simulink model "blockDiagramTask6"  (R2025a)
settings: Solver=VariableStepAuto  StartTime=0.0  StopTime=3.10  RelTol=1e-3
InitFcn:
  | run motor_specs.m
model workspace: external: MATLAB File motor_specs.m (data not in the file)
values from neighbouring files (symbols this model uses):
  A6 = [zeros(2) E; ((-inv(inertiaMatrix)) * stiffnessMatrix), ((-inv(inertiaMatrix)) * dampingMatrix)]    [ssAndTF.m]
  B6 = [zeros(2) inv(inertiaMatrix)]'    [ssAndTF.m]
  C6 = [0 1 0 0]    [ssAndTF.m]
  d_j = 1.5    [motor_specs.m]
  K_E = 0.006741/rpm_to_rs    (= 0.0643718082829)    [motor_specs.m]
  R = 3.23    [motor_specs.m]
  totalGearRatio = torqueSection2 / (torqueSection1 * totalEfficiency)    [ssAndTF.m]
  U_N = 36    [motor_specs.m]
undefined symbols (not defined in the file or in its folder): A8, delta_ratio, k_j, k_theta, my, r_s, sigbuilder_block, T_thresh_2
libraries: slpidlib x3
settings Model: Creator=josef  LastModifiedBy=lucas

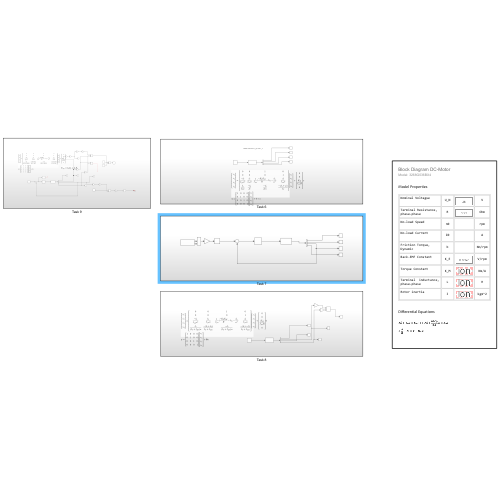
[thumbnail: Simulink's stored preview of the top-level diagram]
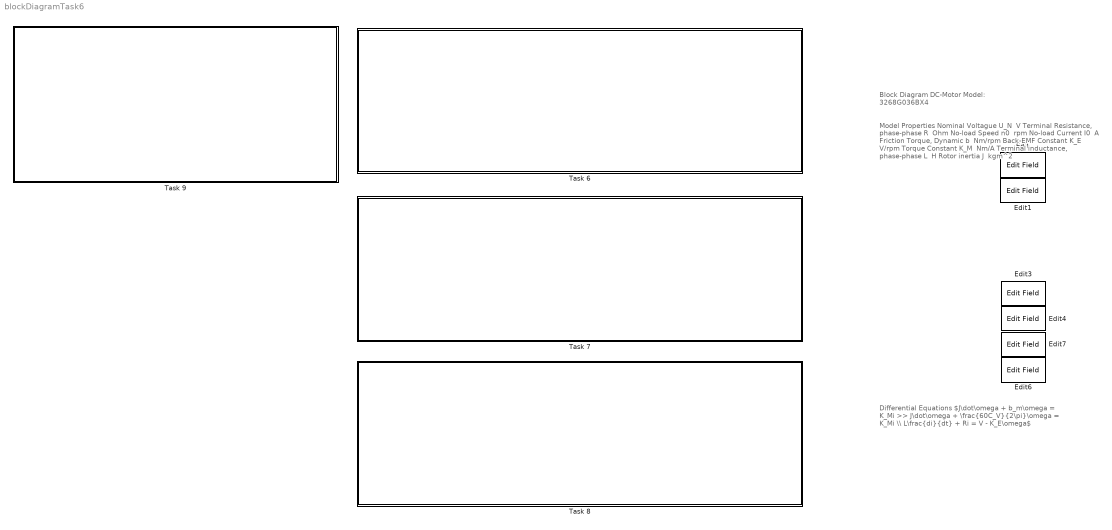
== system blockDiagramTask6 ==
  note: Differential Equations
      |
      | $J\dot\omega + b_m\omega = K_Mi >> J\dot\omega + \frac{60C_V}{2\pi}\omega = K_Mi \\ L\frac{di}{dt} + Ri = V - K_E\omega$
  note: Model Properties
      |
      | Nominal Voltague
      |
      | U_N
      | ​
      | V
      |
      | Terminal Resistance,
      | phase-phase
      | R
      | ​
      | Ohm
      |
      | No-load Speed
      |
      | n0
      | ​
      | rpm
      |
      | No-load Current
      |
      | I0
      | ​
      | A
      |
      | Friction Torque,
      | Dynamic
      | b
      | ​
      | Nm/rpm
      |
      | Back-EMF Constant
      |
      | K_E
      | ​
      | V/rpm
      |
      | Torque Constant
      |
      | K_M
      | ​
      | Nm/A
      |
      | Terminal inductance,
      | phase-phase
      | L
      | ​
      | H
      |
      | Rotor inertia
      |
      | J
      | ​
      | kgm^2
  note: Block Diagram DC-Motor
      | Model: 3268G036BX4
  Edit{,1,3..4,6..7} (6 alike) : EditField  LabelPosition=Hide  ShowInitialText=on  Alignment=Center  Opacity=0
  Task 6 : Subsystem
  Task 7 : Subsystem
  Task 8 : Subsystem
  Task 9 : Subsystem

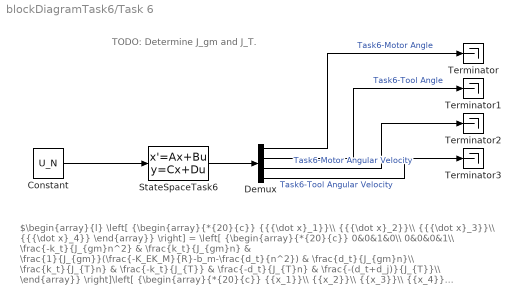
== system blockDiagramTask6/Task 6 ==
  note: TODO: Determine J_gm and J_T.
  note: $\begin{array}{l} \left[ {\begin{array}{*{20}{c}} {{{\dot x}_1}}\\ {{{\dot x}_2}}\\ {{{\dot x}_3}}\\ {{{\dot x}_4}} \end{array}} \right] = \left[ {\begin{array}{*{20}{c}} 0&0&1&0\\ 0&0&0&1\\ \frac{-k_t}{J_{gm}n^2} & \frac{k_t}{J_{gm}n} & \frac{1}{J_{gm}}(\frac{-K_EK_M}{R}-b_m-\frac{d_t}{n^2}) & \frac{d_t}{J_{gm}n}\\ \frac{k_t}{J_{T}n} & \frac{-k_t}{J_{T}} & \frac{-d_t}{J_{T}n} & \frac{-(d_t+d_j)}{J_{T}}\\ \end{array}} \right]\left[ {\begin{array}{*{20}{c}} {{x_1}}\\ {{x_2}}\\ {{x_3}}\\ {{x_4}} \end{array}} \right] + \left[ {\begin{array}{*{20}{c}} 0\\ 0\\ \frac{K_M}{J_{gm}R} \\ 0 \\ \end{array}} \right]u\\ {\bf{y}} = \left[ {\begin{array}{*{20}{c}} 1&0&0&0\\ 0&1&0&0\\ 0&0&1&0\\ 0&0&0&1\\ \end{array}} \right]\left[ {\begin{array}{*{20}{c}} {{x_1}}\\ {{x_2}}\\ {{x_3}}\\ {{x_4}} \end{array}} \right] + 0*u \end{array}$
  Constant : Constant  Value=U_N
  Demux : Demux
  StateSpaceTask6 : StateSpace  A=A6  B=B6  C=C6  D=[0;0;0;0]  InitialCondition=0
  Terminator{,1..3} (4 alike) : Terminator
  wires:
  StateSpaceTask6/1 -> Demux/1
  Demux/1 -> Terminator/1  "Task6-Motor Angle"
  Demux/2 -> Terminator1/1  "Task6-Tool Angle"
  Demux/3 -> Terminator2/1  "Task6-Motor Angular Velocity"
  Demux/4 -> Terminator3/1  "Task6-Tool Angular Velocity"
  Constant/1 -> StateSpaceTask6/1

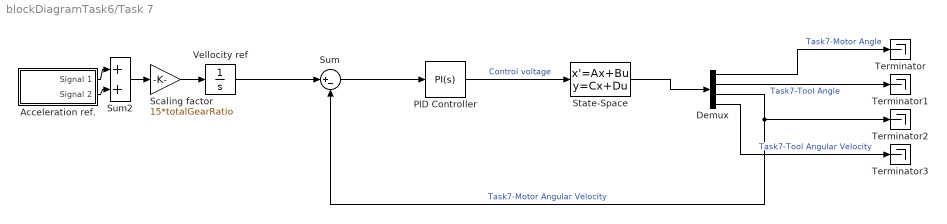
== system blockDiagramTask6/Task 7 ==
  Acceleration ref. : Subsystem  Tag=STV Subsys  LoadFcn=sigbuilder_block('load');  StartFcn=sigbuilder_block('start');  StopFcn=sigbuilder_block('stop');  ClipboardFcn=sigbuilder_block('clipboard');  mask(Sigbuilder block){tuvar=[0:10]}
      mask help: Sigbuilder GUI
      mask init:
      | if ~strcmp(get_param(bdroot(gcbh),'SimulationStatus'),'stopped') tuvar = sigbuilder_block('maskInit'); end
      settings: CopyFcn=sigbuilder_block('copy');  DeleteFcn=sigbuilder_block('delete');  ModelCloseFcn=sigbuilder_block('modelClose');  PreSaveFcn=sigbuilder_block('preSave');  PauseFcn=sigbuilder_block('pause')  ContinueFcn=sigbuilder_block('continue')  NameChangeFcn=sigbuilder_block('namechange');  OpenFcn=sigbuilder_block('open',[210.75 63.75 537 323.25 ]);  CloseFcn=sigbuilder_block('close');
      mask Display: plot(0, 0, 100, 100,[2, 2, 32, 32, 2], [68, 8, 8, 68, 68],[32, 2], [38, 38], [32, 19, 2],[53, 60, 44], [32, 17, 17, 2],[16, 16, 31, 31]);txt = getActiveGroup(gcbh);text(2, 100, txt,'verticalAlignment', 'top');
  Demux : Demux
  PID Controller : slpidlib/PID Controller  Controller=PI  Form=Parallel  TimeDomain=Continuous-time  UseExternalTs=off  SampleTime=-1  IntegratorMethod=Forward Euler  FilterMethod=Forward Euler  ControllerParametersSource=internal  P=0.589073731906208  I=155.603114436522  UseKiTs=off  D=0  UseExternalDerivativeSource=off  N=100  UseFilter=on  TunerSelectOption=Transfer Function Based (PID Tuner App)  InitialConditionSource=internal  InitialConditionForIntegrator=0  InitialConditionForFilter=0  DifferentiatorICPrevScaledInput=0  ExternalReset=none  TrackingMode=off  Kt=1  LimitOutput=off  SatLimitsSource=internal  UpperSaturationLimit=inf  LowerSaturationLimit=-inf  LinearizeAsGain=on  AntiWindupMode=none  Kb=1  LimitIntegrator=off  UpperIntegratorSaturationLimit=inf  LowerIntegratorSaturationLimit=-inf  POutMin=[]  POutMax=[]  IOutMin=[]  IOutMax=[]  DOutMin=[]  DOutMax=[]  NOutMin=[]  NOutMax=[]  SumOutMin=[]  SumOutMax=[]  SaturationOutMin=[]  SaturationOutMax=[]  PParamMin=[]  PParamMax=[]  IParamMin=[]  IParamMax=[]  DParamMin=[]  DParamMax=[]  NParamMin=[]  NParamMax=[]  KbParamMin=[]  KbParamMax=[]  KtParamMin=[]  KtParamMax=[]  KbOutMin=[]  KbOutMax=[]  KtOutMin=[]  KtOutMax=[]  IntegratorOutMin=[]  IntegratorOutMax=[]  FilterOutMin=[]  FilterOutMax=[]  SumI1OutMin=[]  SumI1OutMax=[]  SumI2OutMin=[]  SumI2OutMax=[]  SumI3OutMin=[]  SumI3OutMax=[]  SumI4OutMin=[]  SumI4OutMax=[]  SumDOutMin=[]  SumDOutMax=[]  DifferentiatorOutMin=[]  DifferentiatorOutMax=[]  FilterDiffOutCoefMin=[]  FilterDiffOutCoefMax=[]  ReciprocalOutMin=[]  ReciprocalOutMax=[]  SumDenOutMin=[]  SumDenOutMax=[]  SumNumOutMin=[]  SumNumOutMax=[]  DivideOutMin=[]  DivideOutMax=[]  UdiffTsProdOutMin=[]  UdiffTsProdOutMax=[]  NTsProdOutMin=[]  NTsProdOutMax=[]  UintegralTsProdOutMin=[]  UintegralTsProdOutMax=[]  UngainTsProdOutMin=[]  UngainTsProdOutMax=[]  ClampingZeroOutDataTypeStr=Inherit: Inherit via back propagation  ClampingZeroOutMin=[]  ClampingZeroOutMax=[]  FilterDenConstantOutDataTypeStr=Inherit: Inherit via back propagation  FilterDenConstantOutMin=[]  FilterDenConstantOutMax=[]  PCopyOutDataTypeStr=Inherit: Inherit via back propagation  PCopyOutMin=[]  PCopyOutMax=[]  NCopyOutDataTypeStr=Inherit: Inherit via back propagation  NCopyOutMin=[]  NCopyOutMax=[]  IntegratorContinuousStateAttributes=''  IntegratorStateMustResolveToSignalObject=off  IntegratorRTWStateStorageClass=Auto  FilterContinuousStateAttributes=''  FilterStateMustResolveToSignalObject=off  FilterRTWStateStorageClass=Auto  ParallelPVariant=InternalParameters  IdealPVariant=Disabled  IVariant=InternalParameters  DVariant=Disabled  IntegratorVariant=Continuous  SatVariant=Disabled  AWVariant=Passthrough  PCopyVariant=Disabled  TRVariant=Disabled  FdbkBlocksVariant=Forward  IdealPFdbkVariant=Disabled  SatFdbkVariant=Disabled  DerivativeFilterVariant=Disabled  NVariant=Disabled  NCopyVariant=Disabled_SignalSpec  FilterICVariant=Disabled  IntegratorICVariant=InternalICs  ExternalResetVariant=Disabled  TRSumVariant=Passthrough  SumFdbkVariant=Disabled  SumVariant=Sum_PI  TsampFilterVariant=InternalTs  TsampNgainVariant=Passthrough  TsampIntegralVariant=Disabled_SignalSpec  ExternalSaturationOutDataTypeStr=Inherit: Same as second input  DerivativeSourceVariant=Disabled  PreIntVariant=InternalPreInt
  Scaling factor : Gain  Gain=15*totalGearRatio
  State-Space : StateSpace  A=A6  B=B6  C=C6  D=[0;0;0;0]  InitialCondition=0
  Sum : Sum  Inputs=|+-
  Sum2 : Sum  Inputs=|++
  Terminator{,1..3} (4 alike) : Terminator
  Vellocity ref : Integrator
  wires:
  PID Controller/1 -> State-Space/1  "Control voltage"
  State-Space/1 -> Demux/1
  Demux/1 -> Terminator/1  "Task7-Motor Angle"
  Demux/3 -> Sum/2, Terminator2/1  "Task7-Motor Angular Velocity"
  Demux/4 -> Terminator3/1  "Task7-Tool Angular Velocity"
  Acceleration ref./1(Signal 1) -> Sum2/1
  Acceleration ref./2(Signal 2) -> Sum2/2
  Sum2/1 -> Scaling factor/1
  Scaling factor/1 -> Vellocity ref/1
  Vellocity ref/1 -> Sum/1
  Demux/2 -> Terminator1/1  "Task7-Tool Angle"
  Sum/1 -> PID Controller/1

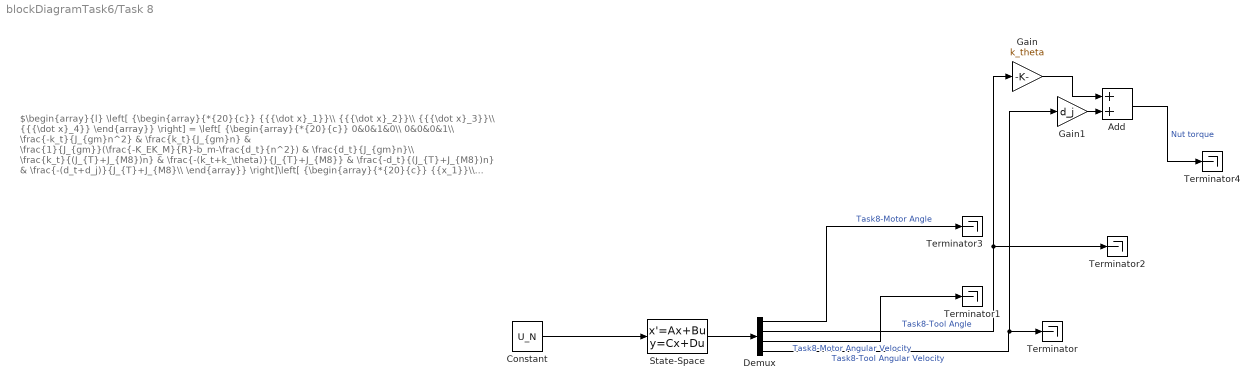
== system blockDiagramTask6/Task 8 ==
  note: $\begin{array}{l} \left[ {\begin{array}{*{20}{c}} {{{\dot x}_1}}\\ {{{\dot x}_2}}\\ {{{\dot x}_3}}\\ {{{\dot x}_4}} \end{array}} \right] = \left[ {\begin{array}{*{20}{c}} 0&0&1&0\\ 0&0&0&1\\ \frac{-k_t}{J_{gm}n^2} & \frac{k_t}{J_{gm}n} & \frac{1}{J_{gm}}(\frac{-K_EK_M}{R}-b_m-\frac{d_t}{n^2}) & \frac{d_t}{J_{gm}n}\\ \frac{k_t}{(J_{T}+J_{M8})n} & \frac{-(k_t+k_\theta)}{J_{T}+J_{M8}} & \frac{-d_t}{(J_{T}+J_{M8})n} & \frac{-(d_t+d_j)}{J_{T}+J_{M8}\\ \end{array}} \right]\left[ {\begin{array}{*{20}{c}} {{x_1}}\\ {{x_2}}\\ {{x_3}}\\ {{x_4}} \end{array}} \right] + \left[ {\begin{array}{*{20}{c}} 0\\ 0\\ \frac{K_M}{J_{gm}R}\\ 0\\ \end{array}} \right]0\\ {\bf{y}} = \left[ {\begin{array}{*{20}{c}} 1&0&0&0\\ 0&1&0&0\\ 0&0&1&0\\ 0&0&0&1\\ \end{array}} \right]\left[ {\begin{array}{*{20}{c}} {{x_1}}\\ {{x_2}}\\ {{x_3}}\\ {{x_4}} \end{array}} \right] + {\bf{0}}u \end{array}$
  Add : Sum
  Constant : Constant  Value=U_N
  Demux : Demux
  Gain : Gain  Gain=k_theta
  Gain1 : Gain  Gain=d_j
  State-Space : StateSpace  A=A8  B=B6  C=C6  D=[0;0;0;0]  InitialCondition=0
  Terminator{,1..4} (5 alike) : Terminator
  wires:
  Constant/1 -> State-Space/1
  State-Space/1 -> Demux/1
  Demux/1 -> Terminator3/1  "Task8-Motor Angle"
  Demux/2 -> Gain/1, Terminator2/1  "Task8-Tool Angle"
  Demux/3 -> Terminator1/1  "Task8-Motor Angular Velocity"
  Demux/4 -> Gain1/1, Terminator/1  "Task8-Tool Angular Velocity"
  Gain1/1 -> Add/2
  Gain/1 -> Add/1
  Add/1 -> Terminator4/1  "Nut torque"

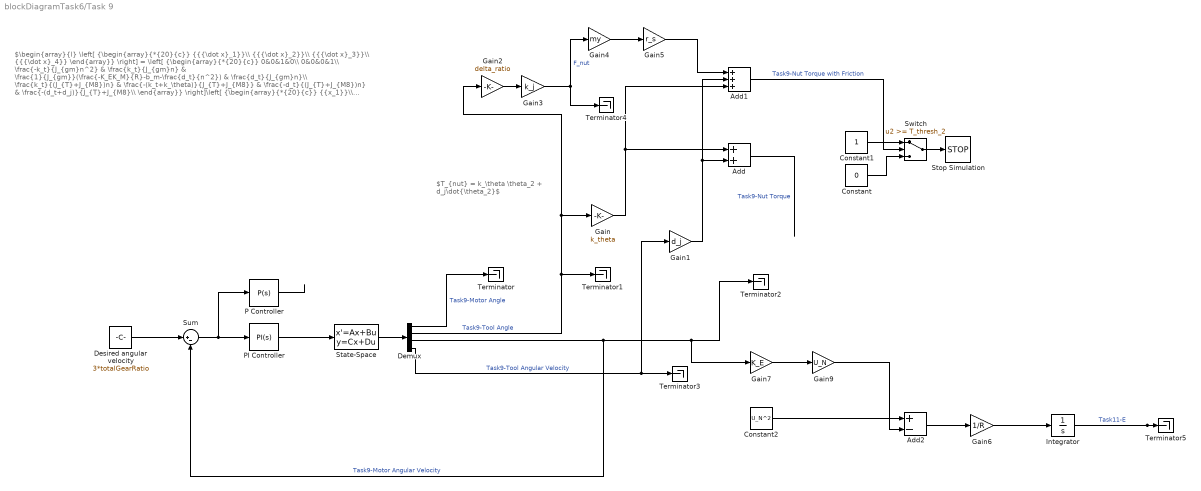
== system blockDiagramTask6/Task 9 ==
  note: $\begin{array}{l} \left[ {\begin{array}{*{20}{c}} {{{\dot x}_1}}\\ {{{\dot x}_2}}\\ {{{\dot x}_3}}\\ {{{\dot x}_4}} \end{array}} \right] = \left[ {\begin{array}{*{20}{c}} 0&0&1&0\\ 0&0&0&1\\ \frac{-k_t}{J_{gm}n^2} & \frac{k_t}{J_{gm}n} & \frac{1}{J_{gm}}(\frac{-K_EK_M}{R}-b_m-\frac{d_t}{n^2}) & \frac{d_t}{J_{gm}n}\\ \frac{k_t}{(J_{T}+J_{M8})n} & \frac{-(k_t+k_\theta)}{J_{T}+J_{M8}} & \frac{-d_t}{(J_{T}+J_{M8})n} & \frac{-(d_t+d_j)}{J_{T}+J_{M8}\\ \end{array}} \right]\left[ {\begin{array}{*{20}{c}} {{x_1}}\\ {{x_2}}\\ {{x_3}}\\ {{x_4}} \end{array}} \right] + \left[ {\begin{array}{*{20}{c}} 0\\ 0\\ \frac{K_M}{J_{gm}R}\\ 0 \\ \end{array}} \right]u\\ {\bf{y}} = \left[ {\begin{array}{*{20}{c}} 1&0&0&0\\ 0&1&0&0\\ 0&0&1&0\\ 0&0&0&1\\ \end{array}} \right]\left[ {\begin{array}{*{20}{c}} {{x_1}}\\ {{x_2}}\\ {{x_3}}\\ {{x_4}} \end{array}} \right] + {\bf{0}}u \end{array}$
  note: $T_{nut} = k_\theta \theta_2 + d_j\dot{\theta_2}$
  Add : Sum
  Add1 : Sum  Inputs=+++
  Add2 : Sum  Inputs=+-
  Constant : Constant  Value=0
  Constant1 : Constant
  Constant2 : Constant  Value=U_N^2
  Demux : Demux
  Desired angular velocity : Constant  Value=3*totalGearRatio
  Gain : Gain  Gain=k_theta
  Gain1 : Gain  Gain=d_j
  Gain2 : Gain  Gain=delta_ratio
  Gain3 : Gain  Gain=k_j
  Gain4 : Gain  Gain=my
  Gain5 : Gain  Gain=r_s
  Gain6 : Gain  Gain=1/R
  Gain7 : Gain  Gain=K_E
  Gain9 : Gain  Gain=U_N
  Integrator : Integrator
  P Controller : slpidlib/PID Controller  Controller=P  Form=Parallel  TimeDomain=Continuous-time  UseExternalTs=off  SampleTime=-1  IntegratorMethod=Forward Euler  FilterMethod=Forward Euler  ControllerParametersSource=internal  P=1  I=1  UseKiTs=off  D=0  UseExternalDerivativeSource=off  N=100  UseFilter=on  TunerSelectOption=Transfer Function Based (PID Tuner App)  InitialConditionSource=internal  InitialConditionForIntegrator=0  InitialConditionForFilter=0  DifferentiatorICPrevScaledInput=0  ExternalReset=none  TrackingMode=off  Kt=1  LimitOutput=off  SatLimitsSource=internal  UpperSaturationLimit=inf  LowerSaturationLimit=-inf  LinearizeAsGain=on  AntiWindupMode=none  Kb=1  LimitIntegrator=off  UpperIntegratorSaturationLimit=inf  LowerIntegratorSaturationLimit=-inf  POutMin=[]  POutMax=[]  IOutMin=[]  IOutMax=[]  DOutMin=[]  DOutMax=[]  NOutMin=[]  NOutMax=[]  SumOutMin=[]  SumOutMax=[]  SaturationOutMin=[]  SaturationOutMax=[]  PParamMin=[]  PParamMax=[]  IParamMin=[]  IParamMax=[]  DParamMin=[]  DParamMax=[]  NParamMin=[]  NParamMax=[]  KbParamMin=[]  KbParamMax=[]  KtParamMin=[]  KtParamMax=[]  KbOutMin=[]  KbOutMax=[]  KtOutMin=[]  KtOutMax=[]  IntegratorOutMin=[]  IntegratorOutMax=[]  FilterOutMin=[]  FilterOutMax=[]  SumI1OutMin=[]  SumI1OutMax=[]  SumI2OutMin=[]  SumI2OutMax=[]  SumI3OutMin=[]  SumI3OutMax=[]  SumI4OutMin=[]  SumI4OutMax=[]  SumDOutMin=[]  SumDOutMax=[]  DifferentiatorOutMin=[]  DifferentiatorOutMax=[]  FilterDiffOutCoefMin=[]  FilterDiffOutCoefMax=[]  ReciprocalOutMin=[]  ReciprocalOutMax=[]  SumDenOutMin=[]  SumDenOutMax=[]  SumNumOutMin=[]  SumNumOutMax=[]  DivideOutMin=[]  DivideOutMax=[]  UdiffTsProdOutMin=[]  UdiffTsProdOutMax=[]  NTsProdOutMin=[]  NTsProdOutMax=[]  UintegralTsProdOutMin=[]  UintegralTsProdOutMax=[]  UngainTsProdOutMin=[]  UngainTsProdOutMax=[]  ClampingZeroOutDataTypeStr=Inherit: Inherit via back propagation  ClampingZeroOutMin=[]  ClampingZeroOutMax=[]  FilterDenConstantOutDataTypeStr=Inherit: Inherit via back propagation  FilterDenConstantOutMin=[]  FilterDenConstantOutMax=[]  PCopyOutDataTypeStr=Inherit: Inherit via back propagation  PCopyOutMin=[]  PCopyOutMax=[]  NCopyOutDataTypeStr=Inherit: Inherit via back propagation  NCopyOutMin=[]  NCopyOutMax=[]  IntegratorContinuousStateAttributes=''  IntegratorStateMustResolveToSignalObject=off  IntegratorRTWStateStorageClass=Auto  FilterContinuousStateAttributes=''  FilterStateMustResolveToSignalObject=off  FilterRTWStateStorageClass=Auto  ParallelPVariant=InternalParameters  IdealPVariant=Disabled  IVariant=Disabled  DVariant=Disabled  IntegratorVariant=Disabled  SatVariant=Disabled  AWVariant=Disabled  PCopyVariant=Disabled  TRVariant=Disabled  FdbkBlocksVariant=Forward  IdealPFdbkVariant=Disabled  SatFdbkVariant=Disabled  DerivativeFilterVariant=Disabled  NVariant=Disabled  NCopyVariant=Disabled_SignalSpec  FilterICVariant=Disabled  IntegratorICVariant=Disabled  ExternalResetVariant=Disabled  TRSumVariant=Passthrough  SumFdbkVariant=Disabled  SumVariant=Passthrough_P  TsampFilterVariant=InternalTs  TsampNgainVariant=Passthrough  TsampIntegralVariant=Disabled_SignalSpec  ExternalSaturationOutDataTypeStr=Inherit: Same as second input  DerivativeSourceVariant=Disabled  PreIntVariant=InternalPreInt
  PI Controller : slpidlib/PID Controller  Controller=PI  Form=Parallel  TimeDomain=Continuous-time  UseExternalTs=off  SampleTime=-1  IntegratorMethod=Forward Euler  FilterMethod=Forward Euler  ControllerParametersSource=internal  P=0  I=13.2590415102096  UseKiTs=off  D=0  UseExternalDerivativeSource=off  N=100  UseFilter=on  TunerSelectOption=Transfer Function Based (PID Tuner App)  InitialConditionSource=internal  InitialConditionForIntegrator=0  InitialConditionForFilter=0  DifferentiatorICPrevScaledInput=0  ExternalReset=none  TrackingMode=off  Kt=1  LimitOutput=off  SatLimitsSource=internal  UpperSaturationLimit=inf  LowerSaturationLimit=-inf  LinearizeAsGain=on  AntiWindupMode=none  Kb=1  LimitIntegrator=off  UpperIntegratorSaturationLimit=inf  LowerIntegratorSaturationLimit=-inf  POutMin=[]  POutMax=[]  IOutMin=[]  IOutMax=[]  DOutMin=[]  DOutMax=[]  NOutMin=[]  NOutMax=[]  SumOutMin=[]  SumOutMax=[]  SaturationOutMin=[]  SaturationOutMax=[]  PParamMin=[]  PParamMax=[]  IParamMin=[]  IParamMax=[]  DParamMin=[]  DParamMax=[]  NParamMin=[]  NParamMax=[]  KbParamMin=[]  KbParamMax=[]  KtParamMin=[]  KtParamMax=[]  KbOutMin=[]  KbOutMax=[]  KtOutMin=[]  KtOutMax=[]  IntegratorOutMin=[]  IntegratorOutMax=[]  FilterOutMin=[]  FilterOutMax=[]  SumI1OutMin=[]  SumI1OutMax=[]  SumI2OutMin=[]  SumI2OutMax=[]  SumI3OutMin=[]  SumI3OutMax=[]  SumI4OutMin=[]  SumI4OutMax=[]  SumDOutMin=[]  SumDOutMax=[]  DifferentiatorOutMin=[]  DifferentiatorOutMax=[]  FilterDiffOutCoefMin=[]  FilterDiffOutCoefMax=[]  ReciprocalOutMin=[]  ReciprocalOutMax=[]  SumDenOutMin=[]  SumDenOutMax=[]  SumNumOutMin=[]  SumNumOutMax=[]  DivideOutMin=[]  DivideOutMax=[]  UdiffTsProdOutMin=[]  UdiffTsProdOutMax=[]  NTsProdOutMin=[]  NTsProdOutMax=[]  UintegralTsProdOutMin=[]  UintegralTsProdOutMax=[]  UngainTsProdOutMin=[]  UngainTsProdOutMax=[]  ClampingZeroOutDataTypeStr=Inherit: Inherit via back propagation  ClampingZeroOutMin=[]  ClampingZeroOutMax=[]  FilterDenConstantOutDataTypeStr=Inherit: Inherit via back propagation  FilterDenConstantOutMin=[]  FilterDenConstantOutMax=[]  PCopyOutDataTypeStr=Inherit: Inherit via back propagation  PCopyOutMin=[]  PCopyOutMax=[]  NCopyOutDataTypeStr=Inherit: Inherit via back propagation  NCopyOutMin=[]  NCopyOutMax=[]  IntegratorContinuousStateAttributes=''  IntegratorStateMustResolveToSignalObject=off  IntegratorRTWStateStorageClass=Auto  FilterContinuousStateAttributes=''  FilterStateMustResolveToSignalObject=off  FilterRTWStateStorageClass=Auto  ParallelPVariant=InternalParameters  IdealPVariant=Disabled  IVariant=InternalParameters  DVariant=Disabled  IntegratorVariant=Continuous  SatVariant=Disabled  AWVariant=Passthrough  PCopyVariant=Disabled  TRVariant=Disabled  FdbkBlocksVariant=Forward  IdealPFdbkVariant=Disabled  SatFdbkVariant=Disabled  DerivativeFilterVariant=Disabled  NVariant=Disabled  NCopyVariant=Disabled_SignalSpec  FilterICVariant=Disabled  IntegratorICVariant=InternalICs  ExternalResetVariant=Disabled  TRSumVariant=Passthrough  SumFdbkVariant=Disabled  SumVariant=Sum_PI  TsampFilterVariant=InternalTs  TsampNgainVariant=Passthrough  TsampIntegralVariant=Disabled_SignalSpec  ExternalSaturationOutDataTypeStr=Inherit: Same as second input  DerivativeSourceVariant=Disabled  PreIntVariant=InternalPreInt
  State-Space : StateSpace  A=A8  B=B6  C=C6  D=[0;0;0;0;]  InitialCondition=0
  Stop Simulation : Stop
  Sum : Sum  Inputs=|+-
  Switch : Switch  Threshold=T_thresh_2  SaturateOnIntegerOverflow=off  InputSameDT=off
  Terminator{,1..5} (6 alike) : Terminator
  wires:
  Constant1/1 -> Switch/1
  Switch/1 -> Stop Simulation/1
  Add/1 -> ?  "Task9-Nut Torque"
  Constant/1 -> Switch/3
  Demux/3 -> Sum/2, Gain7/1, Terminator2/1  "Task9-Motor Angular Velocity"
  Demux/1 -> Terminator/1  "Task9-Motor Angle"
  State-Space/1 -> Demux/1
  Demux/2 -> Terminator1/1, Gain2/1, Gain/1  "Task9-Tool Angle"
  P Controller/1 -> ?
  Demux/4 -> Gain1/1, Terminator3/1  "Task9-Tool Angular Velocity"
  Desired angular velocity/1 -> Sum/1
  Gain1/1 -> Add/2, Add1/2
  Gain/1 -> Add1/3, Add/1
  PI Controller/1 -> State-Space/1
  Sum/1 -> P Controller/1, PI Controller/1
  Gain2/1 -> Gain3/1
  Gain3/1 -> Gain4/1, Terminator4/1  "F_nut"
  Gain4/1 -> Gain5/1
  Gain5/1 -> Add1/1
  Add1/1 -> Switch/2  "Task9-Nut Torque with Friction"
  Constant2/1 -> Add2/1
  Gain9/1 -> Add2/2
  Add2/1 -> Gain6/1
  Gain6/1 -> Integrator/1
  Integrator/1 -> Terminator5/1  "Task11-E"
  Gain7/1 -> Gain9/1

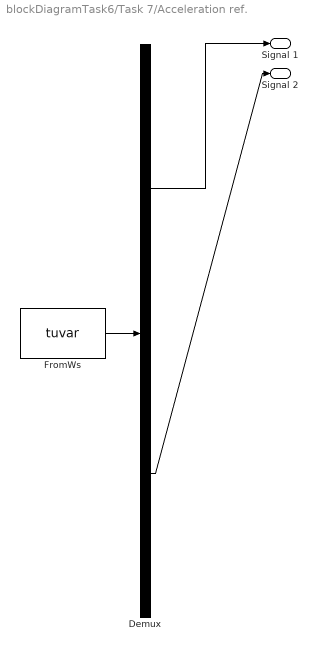
== system blockDiagramTask6/Task 7/Acceleration ref. ==
  Demux : Demux  Tag=STV Demux  Outputs=2
      settings: DisplayOption=none
  FromWs : FromWorkspace  Tag=STV FromWs  VariableName=tuvar
      SigBuilderData=|
      | common.afterFinalStr = 'Extrapolate'
      | common.sampleTime = 0
      | dataSet.timeRange = [0 10]
      | dataSet.name = 'Group 1'
      | sbobj.Groups.Name = 'Group 1'
      | sbobj.Groups.Signals(1).Name = 'Signal 1'
      | sbobj.Groups.Signals(1).XData = [0 0.2 0.2 10]
      | sbobj.Groups.Signals(1).YData = [1 1 0 0]
      | sbobj.Groups.Signals(2).Name = 'Signal 2'
      | sbobj.Groups.Signals(2).XData = [0 2.8 2.8 3 3 10]
      | sbobj.Groups.Signals(2).YData = [0 0 -1 -1 0 0]
  Signal 1 : Outport  Tag=STV Outport
  Signal 2 : Outport  Tag=STV Outport  Port=2
  wires:
  Demux/1 -> Signal 1/1
  FromWs/1 -> Demux/1
  Demux/2 -> Signal 2/1
